simulink model "simulation"  (R2024a)
settings: Solver=ode23tb  StartTime=0.0  StopTime=10  FixedStep=1e-6  RelTol=1e-3
libraries: spsPWMGenerator2LevelLib x2, spsUniversalBridgeLib x2, spsAsynchronousMachineSIUnitsLib x1, spsCurrentMeasurementLib x1, spsPower3phInstantaneousLib x1, spsSeriesRLCBranchLib x1, spsThreePhaseVIMeasurementLib x1, spsThreePhaseSourceLib x1, spsVoltageMeasurementLib x1, sps_lib x1
settings Model: Creator=HP  LastModifiedBy=HP

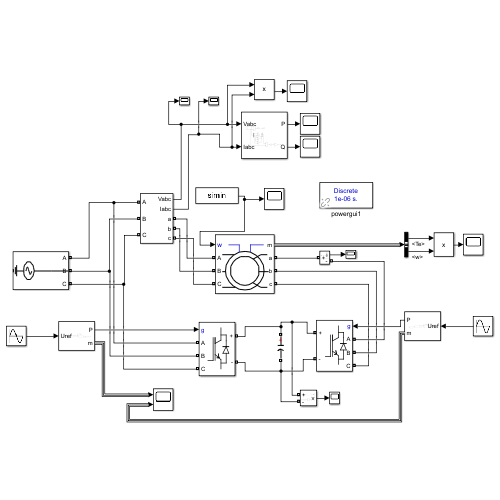
[thumbnail: Simulink's stored preview of the top-level diagram]
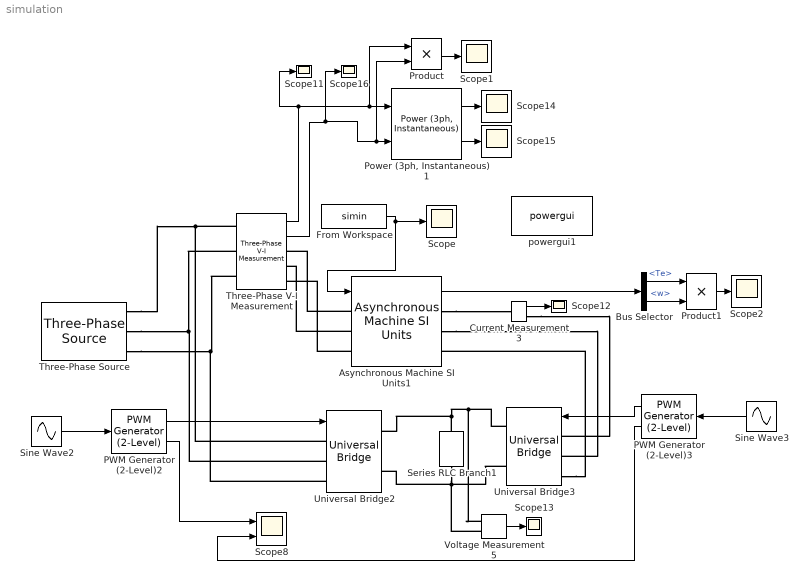
== system simulation ==
  Asynchronous Machine SI Units1 : spsAsynchronousMachineSIUnitsLib/Asynchronous Machine SI Units  RotorType=Wound  PresetModel=No  MechanicalLoad=Speed w  ShowDetailedParameters=on  ReferenceFrame=Rotor  Units=SI  MeasurementBus=on  NominalParameters=[500 100 50]  VoltageRatio=1  Stator=[0.5968 0.0003495]  Rotor=[0.6258 0.005473]  Cage1=[0.4155 0.002066]  Cage2=[0.4168 0.0003495]  Lm=0.0354  Mechanical=[0.05 0.005879 2]  PolePairs=2  InitialConditions=[0 0 0 0 0 0 0 0]  SimulateSaturation=off  Saturation=[14.03593122, 27.81365428, 53.79336849, 72.68890987, 97.98006896, 148.6815601, 215.7428561, 302.9841135, 428.7778367 ; 230, 322, 414, 460, 506, 552, 598, 644, 690]  LoadFlowParameters=1492000  TsPowergui=0  TsBlock=-1  IterativeModel=Trapezoidal non iterative  IterativeDiscreteModel=Trapezoidal non iterative  Pmec=500
  Bus Selector : BusSelector  OutputSignals=Te,w
  Current Measurement3 : spsCurrentMeasurementLib/Current Measurement  PhasorSimulation=off  OutputType=Complex  PSBequivalent=0
  From Workspace : FromWorkspace  VariableName=simin  SampleTime=1e-3  OutputAfterFinalValue=Holding final value
  PWM Generator (2-Level)2 : spsPWMGenerator2LevelLib/PWM Generator (2-Level)  ModulatorType=Three-phase bridge (6 pulses)  ModulatorMode=Unsynchronized  Fc=50*100  Pc=0  nF=27  MinMax="[ -1  1 ]"  SamplingTechnique=Natural  ModulatingSignals=off  m=0.8  Freq=60  Phase=0  Ts=1e-6  ShowCarrierOutport=on
  PWM Generator (2-Level)3 : spsPWMGenerator2LevelLib/PWM Generator (2-Level)  ModulatorType=Three-phase bridge (6 pulses)  ModulatorMode=Unsynchronized  Fc=50*100  Pc=0  nF=27  MinMax="[ -1  1 ]"  SamplingTechnique=Natural  ModulatingSignals=off  m=0.8  Freq=60  Phase=0  Ts=1e-6  ShowCarrierOutport=on
  "Power (3ph, Instantaneous)1" : spsPower3phInstantaneousLib/Power (3ph, Instantaneous)
  Product : Product
  Product1 : Product
  Scope{,1..2,11..16} (9 alike) : Scope
  Scope8 : Scope  NumInputPorts=2
  Series RLC Branch1 : spsSeriesRLCBranchLib/Series RLC Branch  LConnTagsString=__new0  RConnTagsString=__new0  BranchType=C  Resistance=1  Inductance=1e-3  SetiL0=off  InitialCurrent=0  Capacitance=4700e-6  Setx0=off  InitialVoltage=0  Measurements=Branch voltage and current
  Sine Wave2 : Sin  Frequency=2*pi*50  Phase=[0 2*pi/3 -2*pi/3]  SampleTime=0
  Sine Wave3 : Sin  Frequency=2*pi*50  Phase=[0 2*pi/3 -2*pi/3]  SampleTime=0
  Three-Phase V-I Measurement : spsThreePhaseVIMeasurementLib/Three-Phase V-I Measurement  VoltageMeasurement=phase-to-ground  SetLabelV=off  LabelV=Vabc  Vpu=off  VpuLL=off  CurrentMeasurement=yes  SetLabelI=off  LabelI=Iabc  Ipu=off  Pbase=100e6  Vbase=500e3  OutputType=Complex  PhasorSimulation=off  PSBequivalent=0
  Three-Phase Source : spsThreePhaseSourceLib/Three-Phase Source  InternalConnection=Yg  VoltagePhases=off  Voltage=440  PhaseAngle=0  Voltage_phases=[315 315 315]/sqrt(3)  PhaseAngles_phases=[0 -120 +120]  Frequency=50  NonIdealSource=off  SpecifyImpedance=off  Resistance=0.8929  Inductance=16.58e-3  ShortCircuitLevel=100e6  BaseVoltage=25e3  XRratio=7  BusType=swing  Pref=10e3  Qref=0  Prefabc=[10e3, 10e3, 10e3]  Qrefabc=[0, 0, 0]  Qmin=-inf  Qmax=inf
  Universal Bridge2 : spsUniversalBridgeLib/Universal Bridge  Arms=3  SnubberResistance=1e6  SnubberCapacitance=inf  Device=IGBT / Diodes  Ron=1e-3  Lon=0  ForwardVoltages="[  0  0  ]"  ForwardVoltage=0  GTOparameters=[ 10e-6 , 20e-6 ]  IGBTparameters=[ 1e-6 , 2e-6 ]  Measurements=All voltages and currents  Measurements_2=None  converterType=Rectifier
  Universal Bridge3 : spsUniversalBridgeLib/Universal Bridge  Arms=3  SnubberResistance=1e6  SnubberCapacitance=inf  Device=IGBT / Diodes  Ron=1e-3  Lon=0  ForwardVoltages="[  0  0  ]"  ForwardVoltage=0  GTOparameters=[ 10e-6 , 20e-6 ]  IGBTparameters=[ 1e-6 , 2e-6 ]  Measurements=All voltages and currents  Measurements_2=None  converterType=Rectifier
  Voltage Measurement5 : spsVoltageMeasurementLib/Voltage Measurement  PhasorSimulation=off  OutputType=Complex  PSBequivalent=0
  powergui1 : sps_lib/powergui  Priority=1  SimulationMode=Discrete  SampleTime=1e-6  frequency=60  Iterations=50  frequencyindice=50  Pbase=100e6  ErrMax=1e-4  UnitsV=kV  UnitsW=MW  buscounter=0  FunctionMessages=off  echomessages=off  EnableUseOfTLC=off  CurrentSourceSwitches=off  DisableSnubberDevices=off  DisableRonSwitches=off  DisableVfSwitches=off  DisplayEquations=off  AutomaticDiscreteSolvers=off  SolverType=Tustin/Backward Euler (TBE)  Interpol=off  ExternalGateDelay=off  methode=off  Ts=100  x0status=blocks  SPID=on  SwTol=0  HookPort=off  NonlinearTolerance=1e-4  nMaxIteration=100  ContinueOnMaxIteration=off  RestoreLinks=warning  ResistiveCurrentMeasurement=off  Frange=[0:2:500]  Ylog=off  Xlog=on  ShowGrid=off  save=off  variable=ZData  structure=0  ZoomFFT=off  StartTime=0.0  cycles=1  DisplayStyle=1  fundamental=60  FreqAxis=off  MaxFrequency=1000  frequencyindicesteady=1  RmsSteady=1  display=off
  wires:
  PWM Generator (2-Level)3/2 -> Scope8/2
  "Power (3ph, Instantaneous)1"/2 -> Scope15/1
  Voltage Measurement5/1 -> Scope13/1
  Current Measurement3/1 -> Scope12/1
  PWM Generator (2-Level)3/1 -> Universal Bridge3/1
  PWM Generator (2-Level)2/1 -> Universal Bridge2/1
  Three-Phase V-I Measurement/1 -> Scope11/1, Product/1, "Power (3ph, Instantaneous)1"/1
  PWM Generator (2-Level)2/2 -> Scope8/1
  Three-Phase V-I Measurement/2 -> Product/2, "Power (3ph, Instantaneous)1"/2, Scope16/1
  "Power (3ph, Instantaneous)1"/1 -> Scope14/1
  Sine Wave2/1 -> PWM Generator (2-Level)2/1
  From Workspace/1 -> Scope/1, Asynchronous Machine SI Units1/1
  Product/1 -> Scope1/1
  Sine Wave3/1 -> PWM Generator (2-Level)3/1
  Asynchronous Machine SI Units1/1 -> Bus Selector/1
  Bus Selector/2 -> Product1/2  "<w>"
  Bus Selector/1 -> Product1/1  "<Te>"
  Product1/1 -> Scope2/1
  connections:
  Universal Bridge2/RConn1 -- Universal Bridge3/RConn1 -- Voltage Measurement5/LConn1 -- Series RLC Branch1/LConn1
  Universal Bridge2/LConn2 -- Three-Phase Source/RConn2 -- Three-Phase V-I Measurement/LConn2
  Universal Bridge3/RConn2 -- Universal Bridge2/RConn2 -- Series RLC Branch1/RConn1 -- Voltage Measurement5/LConn2
  Universal Bridge3/LConn3 -- Asynchronous Machine SI Units1/RConn3
  Asynchronous Machine SI Units1/RConn1 -- Current Measurement3/LConn1
  Three-Phase V-I Measurement/LConn1 -- Three-Phase Source/RConn1 -- Universal Bridge2/LConn1
  Asynchronous Machine SI Units1/LConn1 -- Three-Phase V-I Measurement/RConn1
  Asynchronous Machine SI Units1/LConn2 -- Three-Phase V-I Measurement/RConn2
  Asynchronous Machine SI Units1/LConn3 -- Three-Phase V-I Measurement/RConn3
  Three-Phase V-I Measurement/LConn3 -- Three-Phase Source/RConn3 -- Universal Bridge2/LConn3
  Current Measurement3/RConn1 -- Universal Bridge3/LConn1
  Asynchronous Machine SI Units1/RConn2 -- Universal Bridge3/LConn2
